simulink model "test_rapidaccel"  (Simulink 7.8)
settings: Solver=ode4  StartTime=0.0  StopTime=100000  FixedStep=0.1  RelTol=1e-3
settings Model: Creator=kkamiya  LastModifiedBy=kkamiya  SimulationMode=rapid-accelerator
settings SFSimCC: SimUserSources=|
  | sfunc_nrlmsise00_wrapper.c
  | nrlmsise-00.c
  | nrlmsise-00_data.c

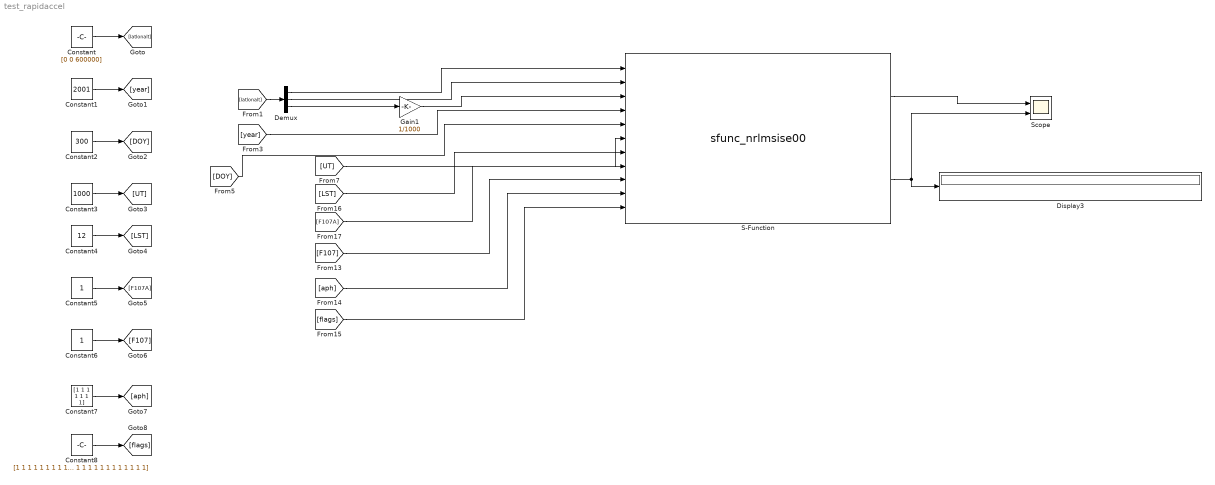
== system test_rapidaccel ==
  Constant : Constant  Value=[0 0 600000]
  Constant1 : Constant  Value=2001
  Constant2 : Constant  Value=300
  Constant3 : Constant  Value=1000
  Constant4 : Constant  Value=12
  Constant5 : Constant
  Constant6 : Constant
  Constant7 : Constant  Value=[1 1 1 1 1 1 1]
  Constant8 : Constant  Value=[1 1 1 1 1 1 1 1 1 1 1 1 1 1 1 1 1 1 1 1 1 1 1]
  Demux : Demux  Outputs=3
  Display3 : Display
      settings: Format=long_e
  Gain1 : Gain  Gain=1/1000
  S-Function : S-Function  FunctionName=sfunc_nrlmsise00  EnableBusSupport=off
  Scope : Scope  NumInputPorts=2
      settings: YMin=442.32~2.752e-018  YMax=442.32~2.752e-018
  wires:
  Constant/1 -> [latlonalt]
  Constant1/1 -> [year]
  Constant2/1 -> [DOY]
  Constant3/1 -> [UT]
  Constant4/1 -> [LST]
  Constant5/1 -> [F107A]
  Constant6/1 -> [F107]
  Constant7/1 -> [aph]
  Constant8/1 -> [flags]
  [latlonalt] -> Demux/1
  Demux/1 -> S-Function/1
  Demux/2 -> S-Function/2
  Demux/3 -> Gain1/1
  [year] -> S-Function/4
  [DOY] -> S-Function/5
  [UT] -> S-Function/6
  [LST] -> S-Function/7
  [F107A] -> S-Function/8
  [F107] -> S-Function/9
  [aph] -> S-Function/10
  [flags] -> S-Function/11
  Gain1/1 -> S-Function/3
  S-Function/2 -> Display3/1, Scope/2
  S-Function/1 -> Scope/1
